simulink model "genericEE"  (R2021a)
settings: Solver=ode8  StartTime=0.0  StopTime=inf  FixedStep=0.001  RelTol=1e-3  EnableMultiTasking=on
StartFcn:
  | addpath('C:\Stud\Mgr_work\casadi-windows-matlabR2016a-v3.5.5')
  | import casadi.*
libraries: CarMaker4SL x35, simulink x1
(part 2 of 3)

== system genericEE/CarMaker/IPG Vehicle/CarAndTrailer/Forces/Tires ==
  note: The TireXX_Out signals will only be used if FileIdent is "CarMaker-Tire-CM4SL" in the tire parameter file!
      | An example parameter file can be found in Data/Tire/DT_CM4SL_UserTire.
  Sync_In : Inport
  TireFL_In : Inport  Port=2
  TireFR_In : Inport  Port=3
  TireRL_In : Inport  Port=4
  TireRR_In : Inport  Port=5
  Bus Creator{1..4} (4 alike) : BusCreator  Inputs=11
  Demux{1..3,8} (4 alike) : Demux  Outputs=7
      settings: DisplayOption=none
  TireFL : Subsystem
  TireFR : Subsystem
  TireRL : Subsystem
  TireRR : Subsystem
  TireFL_Out : Outport
  TireFR_Out : Outport  Port=2
  TireRL_Out : Outport  Port=3
  TireRR_Out : Outport  Port=4
  wires:
  Sync_In/1 -> TireRR/1(Sync_In), TireRL/1(Sync_In), TireFR/1(Sync_In), TireFL/1(Sync_In)
  Bus Creator4/1 -> TireRR_Out/1
  Bus Creator2/1 -> TireRL_Out/1
  Bus Creator1/1 -> TireFR_Out/1
  Demux3/5 -> TireRR/6(Rim_turnv)  "Tire_In Rim_turnv"
  Demux3/4 -> TireRR/5(Rim_rotv)  "Tire_In Rim_rotv"
  Demux3/1 -> TireRR/2(Load)  "Tire_In Load"
  Demux3/7 -> TireRR/8(muRoad)  "Tire_In mu"
  Demux3/6 -> TireRR/7(InclinAngle)  "Tire_In Camber"
  Demux3/2 -> TireRR/3(vxtrans)  "Tire_In vxtrans"
  Demux3/3 -> TireRR/4(vytrans)  "Tire_In vytrans"
  TireRR/11(AlignTrq) -> Bus Creator4/11  "Tire_Out AlignTrq"
  TireRR/10(RollResist) -> Bus Creator4/10  "Tire_Out RollResist"
  TireRR/9(OverturnTrq) -> Bus Creator4/9  "Tire_Out OverturnTrq"
  TireRR/8(LoadFrc) -> Bus Creator4/8  "Tire_Out LoadFrc"
  TireRR/7(SideFrc) -> Bus Creator4/7  "Tire_Out SideFrc"
  TireRR/6(LongFrc) -> Bus Creator4/6  "Tire_Out LongFrc"
  TireRR/5(vBelt) -> Bus Creator4/5  "Tire_Out vBelt"
  TireRR/4(rBelt_eff) -> Bus Creator4/4  "Tire_Out rBelt_eff"
  TireRR/3(TurnSlp) -> Bus Creator4/3  "Tire_Out TurnSlp"
  TireRR/1(Slp) -> Bus Creator4/1  "Tire_Out Slp"
  TireRR/2(Alpha) -> Bus Creator4/2  "Tire_Out Alpha"
  Demux2/5 -> TireRL/6(Rim_turnv)  "Tire_In Rim_turnv"
  Demux2/4 -> TireRL/5(Rim_rotv)  "Tire_In Rim_rotv"
  Demux2/1 -> TireRL/2(Load)  "Tire_In Load"
  Demux2/7 -> TireRL/8(muRoad)  "Tire_In mu"
  Demux2/6 -> TireRL/7(InclinAngle)  "Tire_In Camber"
  Demux2/2 -> TireRL/3(vxtrans)  "Tire_In vxtrans"
  Demux2/3 -> TireRL/4(vytrans)  "Tire_In vytrans"
  TireRL/11(AlignTrq) -> Bus Creator2/11  "Tire_Out AlignTrq"
  TireRL/10(RollResist) -> Bus Creator2/10  "Tire_Out RollResist"
  TireRL/9(OverturnTrq) -> Bus Creator2/9  "Tire_Out OverturnTrq"
  TireRL/8(LoadFrc) -> Bus Creator2/8  "Tire_Out LoadFrc"
  TireRL/7(SideFrc) -> Bus Creator2/7  "Tire_Out SideFrc"
  TireRL/6(LongFrc) -> Bus Creator2/6  "Tire_Out LongFrc"
  TireRL/5(vBelt) -> Bus Creator2/5  "Tire_Out vBelt"
  TireRL/4(rBelt_eff) -> Bus Creator2/4  "Tire_Out rBelt_eff"
  TireRL/3(TurnSlp) -> Bus Creator2/3  "Tire_Out TurnSlp"
  TireRL/1(Slp) -> Bus Creator2/1  "Tire_Out Slp"
  TireRL/2(Alpha) -> Bus Creator2/2  "Tire_Out Alpha"
  Demux1/5 -> TireFR/6(Rim_turnv)  "Tire_In Rim_turnv"
  Demux1/4 -> TireFR/5(Rim_rotv)  "Tire_In Rim_rotv"
  Demux1/1 -> TireFR/2(Load)  "Tire_In Load"
  Demux1/7 -> TireFR/8(muRoad)  "Tire_In mu"
  Demux1/6 -> TireFR/7(InclinAngle)  "Tire_In Camber"
  Demux1/2 -> TireFR/3(vxtrans)  "Tire_In vxtrans"
  Demux1/3 -> TireFR/4(vytrans)  "Tire_In vytrans"
  TireFR/11(AlignTrq) -> Bus Creator1/11  "Tire_Out AlignTrq"
  TireFR/10(RollResist) -> Bus Creator1/10  "Tire_Out RollResist"
  TireFR/9(OverturnTrq) -> Bus Creator1/9  "Tire_Out OverturnTrq"
  TireFR/8(LoadFrc) -> Bus Creator1/8  "Tire_Out LoadFrc"
  TireFR/7(SideFrc) -> Bus Creator1/7  "Tire_Out SideFrc"
  TireFR/6(LongFrc) -> Bus Creator1/6  "Tire_Out LongFrc"
  TireFR/5(vBelt) -> Bus Creator1/5  "Tire_Out vBelt"
  TireFR/4(rBelt_eff) -> Bus Creator1/4  "Tire_Out rBelt_eff"
  TireFR/3(TurnSlp) -> Bus Creator1/3  "Tire_Out TurnSlp"
  TireFR/1(Slp) -> Bus Creator1/1  "Tire_Out Slp"
  TireFR/2(Alpha) -> Bus Creator1/2  "Tire_Out Alpha"
  Demux8/5 -> TireFL/6(Rim_turnv)  "Tire_In Rim_turnv"
  Demux8/4 -> TireFL/5(Rim_rotv)  "Tire_In Rim_rotv"
  TireFL_In/1 -> Demux8/1
  Demux8/1 -> TireFL/2(Load)  "Tire_In Load"
  Demux8/7 -> TireFL/8(muRoad)  "Tire_In mu"
  Demux8/6 -> TireFL/7(InclinAngle)  "Tire_In Camber"
  Demux8/2 -> TireFL/3(vxtrans)  "Tire_In vxtrans"
  Demux8/3 -> TireFL/4(vytrans)  "Tire_In vytrans"
  TireFL/11(AlignTrq) -> Bus Creator3/11  "Tire_Out AlignTrq"
  TireFL/10(RollResist) -> Bus Creator3/10  "Tire_Out RollResist"
  TireFL/9(OverturnTrq) -> Bus Creator3/9  "Tire_Out OverturnTrq"
  TireFL/8(LoadFrc) -> Bus Creator3/8  "Tire_Out LoadFrc"
  TireFL/7(SideFrc) -> Bus Creator3/7  "Tire_Out SideFrc"
  TireFL/6(LongFrc) -> Bus Creator3/6  "Tire_Out LongFrc"
  TireFL/5(vBelt) -> Bus Creator3/5  "Tire_Out vBelt"
  TireFL/4(rBelt_eff) -> Bus Creator3/4  "Tire_Out rBelt_eff"
  TireFL/3(TurnSlp) -> Bus Creator3/3  "Tire_Out TurnSlp"
  TireFL/1(Slp) -> Bus Creator3/1  "Tire_Out Slp"
  TireFL/2(Alpha) -> Bus Creator3/2  "Tire_Out Alpha"
  Bus Creator3/1 -> TireFL_Out/1
  TireFR_In/1 -> Demux1/1
  TireRL_In/1 -> Demux2/1
  TireRR_In/1 -> Demux3/1

== system genericEE/CarMaker/IPG Vehicle/CarAndTrailer/Forces/Vehicle Forces ==
  Sync_In : Inport
  Bus Creator1 : BusCreator  Inputs=12
  Bus Creator8 : BusCreator  Inputs=16
  BusCreator1 : BusCreator  Inputs=4
  BusCreator2 : BusCreator  Inputs=9
  Demux : Demux  Outputs=16
      settings: DisplayOption=none
  Demux1 : Demux  Outputs=12
      settings: DisplayOption=none
  Demux2 : Demux  Outputs=13
      settings: DisplayOption=none
  Forces : S-Function  FunctionName=CM_Sfun  Parameters='Forces'  SFunctionDeploymentMode=off  EnableBusSupport=off
  Terminator : Terminator
  Sync_Out : Outport
  Car.Virtual : Outport  Port=2
  Car.Aero : Outport  Port=3
  Car.Load : Outport  Port=4
  wires:
  BusCreator1/1 -> Terminator/1  "Aero IF (in)"
  Demux2/13 -> BusCreator2/9  "car Aero Trq_1 z"
  Demux2/12 -> BusCreator2/8  "car Aero Trq_1 y"
  Demux2/11 -> BusCreator2/7  "car Aero Trq_1 x"
  Demux2/10 -> BusCreator2/6  "car Aero Frc_1 z"
  Demux2/9 -> BusCreator2/5  "car Aero Frc_1 y"
  Demux2/8 -> BusCreator2/4  "car Aero Frc_1 x"
  Demux2/7 -> BusCreator2/3  "car Aero PoA_1 z"
  Demux2/6 -> BusCreator2/2  "car Aero PoA_1 y"
  Demux2/5 -> BusCreator2/1  "car Aero PoA_1 x"
  Demux2/4 -> BusCreator1/4  "car Aero tau_1"
  Demux2/3 -> BusCreator1/3  "car Aero ApproachVel_1 z"
  Demux2/2 -> BusCreator1/2  "car Aero ApproachVel_1 y"
  Demux2/1 -> BusCreator1/1  "car Aero ApproachVel_1 x"
  Demux/16 -> Bus Creator8/16  "Car Load_3 tz"
  Demux/15 -> Bus Creator8/15  "Car Load_3 ty"
  Demux/14 -> Bus Creator8/14  "Car Load_3 tx"
  Demux/13 -> Bus Creator8/13  "Car Load_3 mass"
  Demux1/12 -> Bus Creator1/12  "Car Virtual Trq_0 z"
  Demux1/11 -> Bus Creator1/11  "Car Virtual Trq_0 y"
  Demux1/10 -> Bus Creator1/10  "Car Virtual Trq_0 x"
  Demux1/9 -> Bus Creator1/9  "Car Virtual Trq_1 z"
  Demux1/8 -> Bus Creator1/8  "Car Virtual Trq_1 y"
  Demux1/7 -> Bus Creator1/7  "Car Virtual Trq_1 x"
  Demux1/6 -> Bus Creator1/6  "Car Virtual Frc_0 z"
  Demux1/5 -> Bus Creator1/5  "Car Virtual Frc_0 y"
  Demux1/4 -> Bus Creator1/4  "Car Virtual Frc_0 x"
  Sync_In/1 -> Forces/1
  Forces/1 -> Sync_Out/1
  BusCreator2/1 -> Car.Aero/1
  Demux1/1 -> Bus Creator1/1  "Car Virtual Frc_1 x"
  Demux1/2 -> Bus Creator1/2  "Car Virtual Frc_1 y"
  Demux1/3 -> Bus Creator1/3  "Car Virtual Frc_1 z"
  Forces/3 -> Demux2/1
  Forces/2 -> Demux1/1
  Bus Creator1/1 -> Car.Virtual/1
  Bus Creator8/1 -> Car.Load/1
  Demux/1 -> Bus Creator8/1  "Car Load_0 mass"
  Demux/2 -> Bus Creator8/2  "Car Load_0 tx"
  Demux/3 -> Bus Creator8/3  "Car Load_0 ty"
  Demux/4 -> Bus Creator8/4  "Car Load_0 tz"
  Demux/5 -> Bus Creator8/5  "Car Load_1 mass"
  Demux/6 -> Bus Creator8/6  "Car Load_1 tx"
  Demux/7 -> Bus Creator8/7  "Car Load_1 ty"
  Demux/8 -> Bus Creator8/8  "Car Load_1 tz"
  Demux/9 -> Bus Creator8/9  "Car Load_2 mass"
  Demux/10 -> Bus Creator8/10  "Car Load_2 tx"
  Demux/11 -> Bus Creator8/11  "Car Load_2 ty"
  Demux/12 -> Bus Creator8/12  "Car Load_2 tz"
  Forces/4 -> Demux/1

== system genericEE/CarMaker/IPG Vehicle/CarAndTrailer/Trailer/CreateBus Car.Hitch.FrcTrq ==
  In1 : Inport
  Bus Creator7 : BusCreator  Inputs=6
  Demux7 : Demux  Outputs=6
      settings: DisplayOption=none
  Out1 : Outport
  wires:
  In1/1 -> Demux7/1
  Bus Creator7/1 -> Out1/1
  Demux7/6 -> Bus Creator7/6  "Car Hitch Trq2Car z"
  Demux7/5 -> Bus Creator7/5  "Car Hitch Trq2Car y"
  Demux7/4 -> Bus Creator7/4  "Car Hitch Trq2Car x"
  Demux7/3 -> Bus Creator7/3  "Car Hitch Frc2Car z"
  Demux7/2 -> Bus Creator7/2  "Car Hitch Frc2Car y"
  Demux7/1 -> Bus Creator7/1  "Car Hitch Frc2Car x"

== system genericEE/CarMaker/IPG Vehicle/CarAndTrailer/Trailer/CreateBus Vhcl.Motion ==
  In1 : Inport
  BusCreator : BusCreator  Inputs=15
  Demux : Demux  Outputs=15
      settings: DisplayOption=none
  Out1 : Outport
  wires:
  Demux/15 -> BusCreator/15  "Vhcl YawAcc"
  Demux/14 -> BusCreator/14  "Vhcl YawVel"
  Demux/13 -> BusCreator/13  "Vhcl Yaw"
  Demux/12 -> BusCreator/12  "Vhcl PitchAcc"
  Demux/11 -> BusCreator/11  "Vhcl PitchVel"
  Demux/10 -> BusCreator/10  "Vhcl Pitch"
  Demux/9 -> BusCreator/9  "Vhcl RollAcc"
  Demux/8 -> BusCreator/8  "Vhcl RollVel"
  Demux/7 -> BusCreator/7  "Vhcl Roll"
  Demux/6 -> BusCreator/6  "Vhcl Hitch_Pos z"
  Demux/5 -> BusCreator/5  "Vhcl Hitch_Pos y"
  Demux/4 -> BusCreator/4  "Vhcl Hitch_Pos x"
  Demux/3 -> BusCreator/3  "Vhcl sRoad"
  Demux/2 -> BusCreator/2  "Vhcl Distance"
  Demux/1 -> BusCreator/1  "Vhcl v"
  In1/1 -> Demux/1
  BusCreator/1 -> Out1/1

== system genericEE/CarMaker/IPG Vehicle/CarAndTrailer/Trailer/CreateBus Vhcl.PoI ==
  In1 : Inport
  Bus Creator3 : BusCreator  Inputs=18
  Demux3 : Demux  Outputs=18
      settings: DisplayOption=none
  Out1 : Outport
  wires:
  Demux3/18 -> Bus Creator3/18  "Vhcl PoI_GCS Elev"
  Demux3/17 -> Bus Creator3/17  "Vhcl PoI_GCS Lat"
  Demux3/16 -> Bus Creator3/16  "Vhcl PoI_GCS Long"
  Demux3/15 -> Bus Creator3/15  "Vhcl PoI_Acc_1 z"
  Demux3/14 -> Bus Creator3/14  "Vhcl PoI_Acc_1 y"
  Demux3/13 -> Bus Creator3/13  "Vhcl PoI_Acc_1 x"
  Demux3/12 -> Bus Creator3/12  "Vhcl PoI_Vel_1 z"
  Demux3/11 -> Bus Creator3/11  "Vhcl PoI_Vel_1 y"
  Demux3/10 -> Bus Creator3/10  "Vhcl PoI_Vel_1 x"
  Demux3/9 -> Bus Creator3/9  "Vhcl PoI_Acc z"
  Demux3/8 -> Bus Creator3/8  "Vhcl PoI_Acc y"
  Demux3/7 -> Bus Creator3/7  "Vhcl PoI_Acc x"
  Demux3/6 -> Bus Creator3/6  "Vhcl PoI_Vel z"
  Demux3/5 -> Bus Creator3/5  "Vhcl PoI_Vel y"
  Demux3/4 -> Bus Creator3/4  "Vhcl PoI_Vel x"
  Demux3/3 -> Bus Creator3/3  "Vhcl PoI_Pos z"
  Demux3/2 -> Bus Creator3/2  "Vhcl PoI_Pos y"
  In1/1 -> Demux3/1
  Bus Creator3/1 -> Out1/1
  Demux3/1 -> Bus Creator3/1  "Vhcl PoI_Pos x"

== system genericEE/CarMaker/IPG Vehicle/CarAndTrailer/Trailer/CreateBus Vhcl.Steering ==
  In1 : Inport
  Bus Creator3 : BusCreator  Inputs=4
  Demux : Demux
      settings: DisplayOption=none
  Out1 : Outport
  wires:
  Bus Creator3/1 -> Out1/1
  Demux/1 -> Bus Creator3/1  "Vhcl Steering Ang"
  Demux/3 -> Bus Creator3/3  "Vhcl Steering AngAcc"
  Demux/2 -> Bus Creator3/2  "Vhcl Steering AngVel"
  Demux/4 -> Bus Creator3/4  "Vhcl Steering Trq"
  In1/1 -> Demux/1

== system genericEE/CarMaker/IPG Vehicle/CarAndTrailer/Trailer/CreateBus Vhcl.Wheel.FL ==
  In1 : Inport
  Bus Creator3 : BusCreator  Inputs=14
  Demux3 : Demux  Outputs=14
      settings: DisplayOption=none
  Out1 : Outport
  wires:
  Demux3/14 -> Bus Creator3/14  "Vhcl Wheel FL Trq_WhlBearing"
  Demux3/13 -> Bus Creator3/13  "Vhcl Wheel FL Trq_T2W"
  Demux3/12 -> Bus Creator3/12  "Vhcl Wheel FL SideSlip"
  Demux3/11 -> Bus Creator3/11  "Vhcl Wheel FL LongSlip"
  Demux3/10 -> Bus Creator3/10  "Vhcl Wheel FL vBelt"
  Demux3/9 -> Bus Creator3/9  "Vhcl Wheel FL Fz"
  Demux3/8 -> Bus Creator3/8  "Vhcl Wheel FL Fy"
  Demux3/7 -> Bus Creator3/7  "Vhcl Wheel FL Fx"
  Demux3/6 -> Bus Creator3/6  "Vhcl Wheel FL r_zxy z"
  Demux3/5 -> Bus Creator3/5  "Vhcl Wheel FL r_zxy y"
  Demux3/4 -> Bus Creator3/4  "Vhcl Wheel FL r_zxy x"
  Demux3/3 -> Bus Creator3/3  "Vhcl Wheel FL t z"
  Demux3/2 -> Bus Creator3/2  "Vhcl Wheel FL t y"
  In1/1 -> Demux3/1
  Bus Creator3/1 -> Out1/1
  Demux3/1 -> Bus Creator3/1  "Vhcl Wheel FL t x"

== system genericEE/CarMaker/IPG Vehicle/CarAndTrailer/Trailer/CreateBus Vhcl.Wheel.FR ==
  In1 : Inport
  Bus Creator3 : BusCreator  Inputs=14
  Demux3 : Demux  Outputs=14
      settings: DisplayOption=none
  Out1 : Outport
  wires:
  Demux3/14 -> Bus Creator3/14  "Vhcl Wheel FR Trq_WhlBearing"
  Demux3/13 -> Bus Creator3/13  "Vhcl Wheel FR Trq_T2W"
  Demux3/12 -> Bus Creator3/12  "Vhcl Wheel FR SideSlip"
  Demux3/11 -> Bus Creator3/11  "Vhcl Wheel FR LongSlip"
  Demux3/10 -> Bus Creator3/10  "Vhcl Wheel FR vBelt"
  Demux3/9 -> Bus Creator3/9  "Vhcl Wheel FR Fz"
  Demux3/8 -> Bus Creator3/8  "Vhcl Wheel FR Fy"
  Demux3/7 -> Bus Creator3/7  "Vhcl Wheel FR Fx"
  Demux3/6 -> Bus Creator3/6  "Vhcl Wheel FR r_zxy z"
  Demux3/5 -> Bus Creator3/5  "Vhcl Wheel FR r_zxy y"
  Demux3/4 -> Bus Creator3/4  "Vhcl Wheel FR r_zxy x"
  Demux3/3 -> Bus Creator3/3  "Vhcl Wheel FR t z"
  Demux3/2 -> Bus Creator3/2  "Vhcl Wheel FR t y"
  In1/1 -> Demux3/1
  Bus Creator3/1 -> Out1/1
  Demux3/1 -> Bus Creator3/1  "Vhcl Wheel FR t x"

== system genericEE/CarMaker/IPG Vehicle/CarAndTrailer/Trailer/CreateBus Vhcl.Wheel.RL ==
  In1 : Inport
  Bus Creator3 : BusCreator  Inputs=14
  Demux3 : Demux  Outputs=14
      settings: DisplayOption=none
  Out1 : Outport
  wires:
  Demux3/14 -> Bus Creator3/14  "Vhcl Wheel RL Trq_WhlBearing"
  Demux3/13 -> Bus Creator3/13  "Vhcl Wheel RL Trq_T2W"
  Demux3/12 -> Bus Creator3/12  "Vhcl Wheel RL SideSlip"
  Demux3/11 -> Bus Creator3/11  "Vhcl Wheel RL LongSlip"
  Demux3/10 -> Bus Creator3/10  "Vhcl Wheel RL vBelt"
  Demux3/9 -> Bus Creator3/9  "Vhcl Wheel RL Fz"
  Demux3/8 -> Bus Creator3/8  "Vhcl Wheel RL Fy"
  Demux3/7 -> Bus Creator3/7  "Vhcl Wheel RL Fx"
  Demux3/6 -> Bus Creator3/6  "Vhcl Wheel RL r_zxy z"
  Demux3/5 -> Bus Creator3/5  "Vhcl Wheel RL r_zxy y"
  Demux3/4 -> Bus Creator3/4  "Vhcl Wheel RL r_zxy x"
  Demux3/3 -> Bus Creator3/3  "Vhcl Wheel RL t z"
  Demux3/2 -> Bus Creator3/2  "Vhcl Wheel RL t y"
  In1/1 -> Demux3/1
  Bus Creator3/1 -> Out1/1
  Demux3/1 -> Bus Creator3/1  "Vhcl Wheel RL t x"

== system genericEE/CarMaker/IPG Vehicle/CarAndTrailer/Trailer/CreateBus Vhcl.Wheel.RR ==
  In1 : Inport
  Bus Creator3 : BusCreator  Inputs=14
  Demux3 : Demux  Outputs=14
      settings: DisplayOption=none
  Out1 : Outport
  wires:
  Demux3/14 -> Bus Creator3/14  "Vhcl Wheel RR Trq_WhlBearing"
  Demux3/13 -> Bus Creator3/13  "Vhcl Wheel RR Trq_T2W"
  Demux3/12 -> Bus Creator3/12  "Vhcl Wheel RR SideSlip"
  Demux3/11 -> Bus Creator3/11  "Vhcl Wheel RR LongSlip"
  Demux3/10 -> Bus Creator3/10  "Vhcl Wheel RR vBelt"
  Demux3/9 -> Bus Creator3/9  "Vhcl Wheel RR Fz"
  Demux3/8 -> Bus Creator3/8  "Vhcl Wheel RR Fy"
  Demux3/7 -> Bus Creator3/7  "Vhcl Wheel RR Fx"
  Demux3/6 -> Bus Creator3/6  "Vhcl Wheel RR r_zxy z"
  Demux3/5 -> Bus Creator3/5  "Vhcl Wheel RR r_zxy y"
  Demux3/4 -> Bus Creator3/4  "Vhcl Wheel RR r_zxy x"
  Demux3/3 -> Bus Creator3/3  "Vhcl Wheel RR t z"
  Demux3/2 -> Bus Creator3/2  "Vhcl Wheel RR t y"
  In1/1 -> Demux3/1
  Bus Creator3/1 -> Out1/1
  Demux3/1 -> Bus Creator3/1  "Vhcl Wheel RR t x"

== system genericEE/CarMaker/VehicleControl/CreateBus VhclCtrl/Environmental Envelope Protection/Control switcher with memory ==
  v : Inport
  thr : Inport  Port=2
  Integrator : Integrator  LimitOutput=on  UpperSaturationLimit=0.2  LowerSaturationLimit=-0.2
  MATLAB Function : MATLAB Function  TreatAsAtomicUnit=on
  Scope : Scope  NumInputPorts=2
  Sign : Signum
  control_flag : Outport
  wires:
  Sign/1 -> control_flag/1
  MATLAB Function/1(control_on) -> Scope/1, Integrator/1
  thr/1 -> MATLAB Function/2(thr)
  Integrator/1 -> Scope/2, Sign/1
  v/1 -> MATLAB Function/1(v)

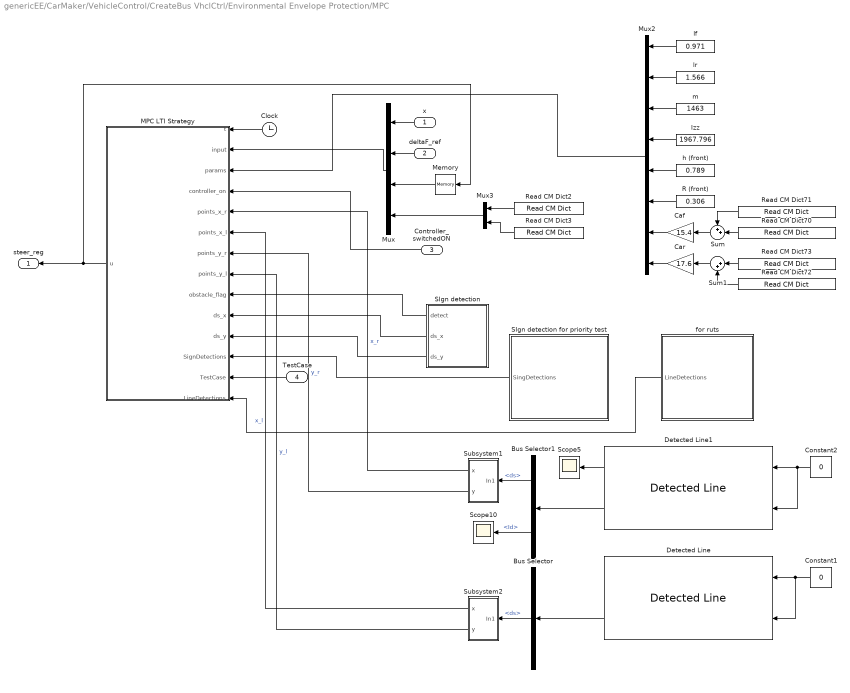
== system genericEE/CarMaker/VehicleControl/CreateBus VhclCtrl/Environmental Envelope Protection/MPC ==
  x : Inport
  deltaF_ref : Inport  Port=2
  Controller_switchedON : Inport  Port=3
  TestCase : Inport  Port=4
  Bus Selector : BusSelector  OutputSignals=ds
  Bus Selector1 : BusSelector  OutputSignals=ds,Id
  Caf : Gain  Gain=15.4
  Car : Gain  Gain=17.6
  Clock : Clock
  Constant1 : Constant  Value=0
  Constant2 : Constant  Value=0
  Detected Line : CarMaker4SL/Sensors/Detected Line  xname=INPORT  xstime=Continuous  xside=left
      settings: SourceProductName=CarMaker4SL
  Detected Line1 : CarMaker4SL/Sensors/Detected Line  xname=INPORT  xstime=Continuous  xside=right
      settings: SourceProductName=CarMaker4SL
  Izz : Constant  Value=1967.796
  MPC LTI Strategy : MATLAB Function  TreatAsAtomicUnit=on  SystemSampleTime=0.05
  Memory : Memory
  Mux : Mux
  Mux2 : Mux  Inputs=8
  Mux3 : Mux  Inputs=2
  R (front) : Constant  Value=0.306
  Read CM Dict2 : CarMaker4SL/Read CM Dict  xname=Car.tx  xsync=off  xstime=Continuous
  Read CM Dict3 : CarMaker4SL/Read CM Dict  xname=Car.ty  xsync=off  xstime=Continuous
  Read CM Dict70 : CarMaker4SL/Read CM Dict  xname=Vhcl.FL.Fz  xsync=off  xstime=Continuous
  Read CM Dict71 : CarMaker4SL/Read CM Dict  xname=Vhcl.FR.Fz  xsync=off  xstime=Continuous
  Read CM Dict72 : CarMaker4SL/Read CM Dict  xname=Vhcl.RL.Fz  xsync=off  xstime=Continuous
  Read CM Dict73 : CarMaker4SL/Read CM Dict  xname=Vhcl.RR.Fz  xsync=off  xstime=Continuous
  SIgn detection : Subsystem
  SIgn detection for priority test : Subsystem
  Scope10 : Scope
  Scope5 : Scope
  Subsystem1 : Subsystem
  Subsystem2 : Subsystem
  Sum : Sum  Inputs=++|
  Sum1 : Sum  Inputs=|++
  for ruts : Subsystem
  h (front) : Constant  Value=0.789
  lf : Constant  Value=0.971
  lr : Constant  Value=1.566
  m : Constant  Value=1463
  steer_reg : Outport  VectorParamsAs1DForOutWhenUnconnected=off
  wires:
  Mux/1 -> MPC LTI Strategy/2(input)
  deltaF_ref/1 -> Mux/2
  x/1 -> Mux/1
  Clock/1 -> MPC LTI Strategy/1(t)
  h (front)/1 -> Mux2/5
  R (front)/1 -> Mux2/6
  Mux2/1 -> MPC LTI Strategy/3(params)
  Izz/1 -> Mux2/4
  m/1 -> Mux2/3
  lr/1 -> Mux2/2
  lf/1 -> Mux2/1
  Read CM Dict71/1 -> Sum/1
  Read CM Dict70/1 -> Sum/2
  Sum/1 -> Caf/1
  Caf/1 -> Mux2/7
  Read CM Dict73/1 -> Sum1/1
  Sum1/1 -> Car/1
  Read CM Dict72/1 -> Sum1/2
  Car/1 -> Mux2/8
  Controller_switchedON/1 -> MPC LTI Strategy/4(controller_on)
  Memory/1 -> Mux/3
  Subsystem1/1(x) -> MPC LTI Strategy/5(points_x_r)  "x_r"
  Subsystem1/2(y) -> MPC LTI Strategy/7(points_y_r)  "y_r"
  Subsystem2/2(y) -> MPC LTI Strategy/8(points_y_l)  "y_l"
  Detected Line/2 -> Bus Selector/1
  Constant2/1 -> Detected Line1/2, Detected Line1/1
  Bus Selector1/1 -> Subsystem1/1(In1)  "<ds>"
  Subsystem2/1(x) -> MPC LTI Strategy/6(points_x_l)  "x_l"
  Constant1/1 -> Detected Line/2, Detected Line/1
  Bus Selector/1 -> Subsystem2/1(In1)  "<ds>"
  Detected Line1/2 -> Bus Selector1/1
  Read CM Dict2/1 -> Mux3/1
  Read CM Dict3/1 -> Mux3/2
  Mux3/1 -> Mux/4
  SIgn detection/1(detect) -> MPC LTI Strategy/9(obstacle_flag)
  SIgn detection/3(ds_y) -> MPC LTI Strategy/11(ds_y)
  SIgn detection/2(ds_x) -> MPC LTI Strategy/10(ds_x)
  Detected Line1/1 -> Scope5/1
  Bus Selector1/2 -> Scope10/1  "<Id>"
  SIgn detection for priority test/1(SingDetections) -> MPC LTI Strategy/12(SignDetections)
  TestCase/1 -> MPC LTI Strategy/13(TestCase)
  for ruts/1(LineDetections) -> MPC LTI Strategy/14(LineDetections)
  MPC LTI Strategy/1(u) -> steer_reg/1, Memory/1

== system genericEE/CarMaker/VehicleControl/CreateBus VhclCtrl/Environmental Envelope Protection/Reference Generator ==
  Clock : Clock
  Clock2 : Clock
  Constant1 : Constant  Value=0
  Gain3 : Gain  Gain=0.1
  Gain4 : Gain  Gain=0.3
  Rate Limiter : RateLimiter  RisingSlewLimit=0.3  FallingSlewLimit=-0.3  SampleTimeMode=inherited
  Sin : Trigonometry
  Switch : Switch  Criteria=u2 > Threshold  Threshold=30
  Out1 : Outport
  wires:
  Clock2/1 -> Gain4/1
  Gain4/1 -> Sin/1
  Rate Limiter/1 -> Out1/1
  Switch/1 -> Rate Limiter/1
  Clock/1 -> Switch/2
  Sin/1 -> Gain3/1
  Gain3/1 -> Switch/3
  Constant1/1 -> Switch/1

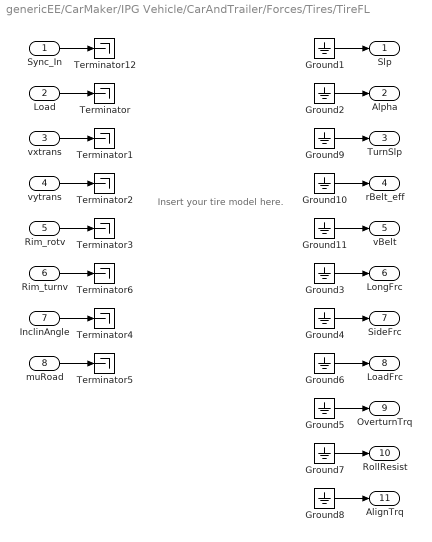
== system genericEE/CarMaker/IPG Vehicle/CarAndTrailer/Forces/Tires/TireFL ==
  note: Insert your tire model here.
  Sync_In : Inport
  Load : Inport  Port=2
  vxtrans : Inport  Port=3
  vytrans : Inport  Port=4
  Rim_rotv : Inport  Port=5
  Rim_turnv : Inport  Port=6
  InclinAngle : Inport  Port=7
  muRoad : Inport  Port=8
  Ground{1..11} (11 alike) : Ground
  Terminator{,1..6,12} (8 alike) : Terminator
  Slp : Outport
  Alpha : Outport  Port=2
  TurnSlp : Outport  Port=3
  rBelt_eff : Outport  Port=4
  vBelt : Outport  Port=5
  LongFrc : Outport  Port=6
  SideFrc : Outport  Port=7
  LoadFrc : Outport  Port=8
  OverturnTrq : Outport  Port=9
  RollResist : Outport  Port=10
  AlignTrq : Outport  Port=11
  wires:
  Ground11/1 -> vBelt/1
  Ground10/1 -> rBelt_eff/1
  Ground9/1 -> TurnSlp/1
  Rim_turnv/1 -> Terminator6/1
  Sync_In/1 -> Terminator12/1
  Ground2/1 -> Alpha/1
  Ground3/1 -> LongFrc/1
  Ground4/1 -> SideFrc/1
  Ground5/1 -> OverturnTrq/1
  vxtrans/1 -> Terminator1/1
  vytrans/1 -> Terminator2/1
  Rim_rotv/1 -> Terminator3/1
  InclinAngle/1 -> Terminator4/1
  muRoad/1 -> Terminator5/1
  Load/1 -> Terminator/1
  Ground1/1 -> Slp/1
  Ground6/1 -> LoadFrc/1
  Ground7/1 -> RollResist/1
  Ground8/1 -> AlignTrq/1

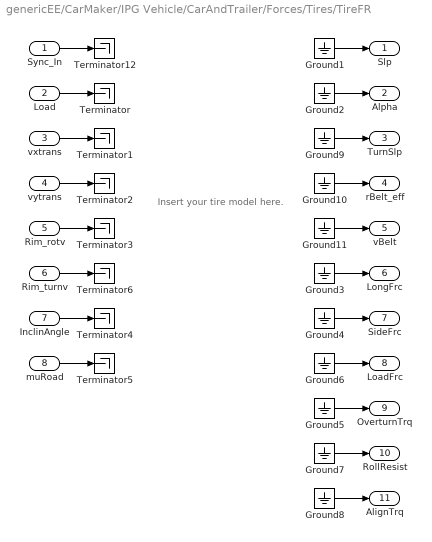
== system genericEE/CarMaker/IPG Vehicle/CarAndTrailer/Forces/Tires/TireFR ==
  note: Insert your tire model here.
  Sync_In : Inport
  Load : Inport  Port=2
  vxtrans : Inport  Port=3
  vytrans : Inport  Port=4
  Rim_rotv : Inport  Port=5
  Rim_turnv : Inport  Port=6
  InclinAngle : Inport  Port=7
  muRoad : Inport  Port=8
  Ground{1..11} (11 alike) : Ground
  Terminator{,1..6,12} (8 alike) : Terminator
  Slp : Outport
  Alpha : Outport  Port=2
  TurnSlp : Outport  Port=3
  rBelt_eff : Outport  Port=4
  vBelt : Outport  Port=5
  LongFrc : Outport  Port=6
  SideFrc : Outport  Port=7
  LoadFrc : Outport  Port=8
  OverturnTrq : Outport  Port=9
  RollResist : Outport  Port=10
  AlignTrq : Outport  Port=11
  wires:
  Ground11/1 -> vBelt/1
  Ground10/1 -> rBelt_eff/1
  Ground9/1 -> TurnSlp/1
  Rim_turnv/1 -> Terminator6/1
  Sync_In/1 -> Terminator12/1
  Ground2/1 -> Alpha/1
  Ground3/1 -> LongFrc/1
  Ground4/1 -> SideFrc/1
  Ground5/1 -> OverturnTrq/1
  vxtrans/1 -> Terminator1/1
  vytrans/1 -> Terminator2/1
  Rim_rotv/1 -> Terminator3/1
  InclinAngle/1 -> Terminator4/1
  muRoad/1 -> Terminator5/1
  Load/1 -> Terminator/1
  Ground1/1 -> Slp/1
  Ground6/1 -> LoadFrc/1
  Ground7/1 -> RollResist/1
  Ground8/1 -> AlignTrq/1

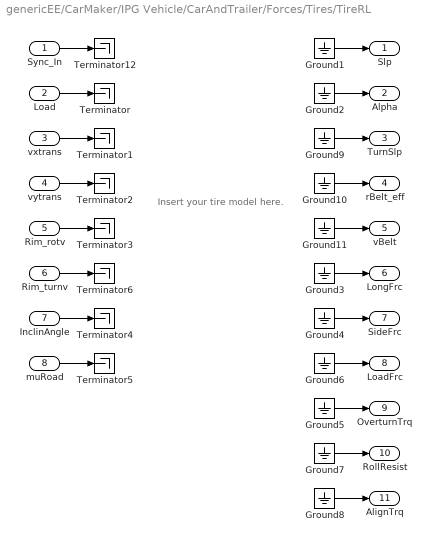
== system genericEE/CarMaker/IPG Vehicle/CarAndTrailer/Forces/Tires/TireRL ==
  note: Insert your tire model here.
  Sync_In : Inport
  Load : Inport  Port=2
  vxtrans : Inport  Port=3
  vytrans : Inport  Port=4
  Rim_rotv : Inport  Port=5
  Rim_turnv : Inport  Port=6
  InclinAngle : Inport  Port=7
  muRoad : Inport  Port=8
  Ground{1..11} (11 alike) : Ground
  Terminator{,1..6,12} (8 alike) : Terminator
  Slp : Outport
  Alpha : Outport  Port=2
  TurnSlp : Outport  Port=3
  rBelt_eff : Outport  Port=4
  vBelt : Outport  Port=5
  LongFrc : Outport  Port=6
  SideFrc : Outport  Port=7
  LoadFrc : Outport  Port=8
  OverturnTrq : Outport  Port=9
  RollResist : Outport  Port=10
  AlignTrq : Outport  Port=11
  wires:
  Ground11/1 -> vBelt/1
  Ground10/1 -> rBelt_eff/1
  Ground9/1 -> TurnSlp/1
  Rim_turnv/1 -> Terminator6/1
  Sync_In/1 -> Terminator12/1
  Ground2/1 -> Alpha/1
  Ground3/1 -> LongFrc/1
  Ground4/1 -> SideFrc/1
  Ground5/1 -> OverturnTrq/1
  vxtrans/1 -> Terminator1/1
  vytrans/1 -> Terminator2/1
  Rim_rotv/1 -> Terminator3/1
  InclinAngle/1 -> Terminator4/1
  muRoad/1 -> Terminator5/1
  Load/1 -> Terminator/1
  Ground1/1 -> Slp/1
  Ground6/1 -> LoadFrc/1
  Ground7/1 -> RollResist/1
  Ground8/1 -> AlignTrq/1

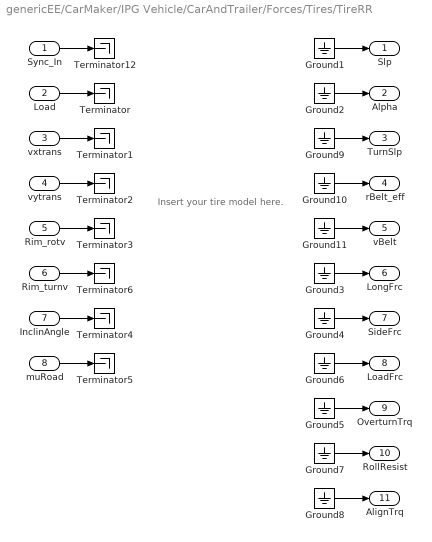
== system genericEE/CarMaker/IPG Vehicle/CarAndTrailer/Forces/Tires/TireRR ==
  note: Insert your tire model here.
  Sync_In : Inport
  Load : Inport  Port=2
  vxtrans : Inport  Port=3
  vytrans : Inport  Port=4
  Rim_rotv : Inport  Port=5
  Rim_turnv : Inport  Port=6
  InclinAngle : Inport  Port=7
  muRoad : Inport  Port=8
  Ground{1..11} (11 alike) : Ground
  Terminator{,1..6,12} (8 alike) : Terminator
  Slp : Outport
  Alpha : Outport  Port=2
  TurnSlp : Outport  Port=3
  rBelt_eff : Outport  Port=4
  vBelt : Outport  Port=5
  LongFrc : Outport  Port=6
  SideFrc : Outport  Port=7
  LoadFrc : Outport  Port=8
  OverturnTrq : Outport  Port=9
  RollResist : Outport  Port=10
  AlignTrq : Outport  Port=11
  wires:
  Ground11/1 -> vBelt/1
  Ground10/1 -> rBelt_eff/1
  Ground9/1 -> TurnSlp/1
  Rim_turnv/1 -> Terminator6/1
  Sync_In/1 -> Terminator12/1
  Ground2/1 -> Alpha/1
  Ground3/1 -> LongFrc/1
  Ground4/1 -> SideFrc/1
  Ground5/1 -> OverturnTrq/1
  vxtrans/1 -> Terminator1/1
  vytrans/1 -> Terminator2/1
  Rim_rotv/1 -> Terminator3/1
  InclinAngle/1 -> Terminator4/1
  muRoad/1 -> Terminator5/1
  Load/1 -> Terminator/1
  Ground1/1 -> Slp/1
  Ground6/1 -> LoadFrc/1
  Ground7/1 -> RollResist/1
  Ground8/1 -> AlignTrq/1

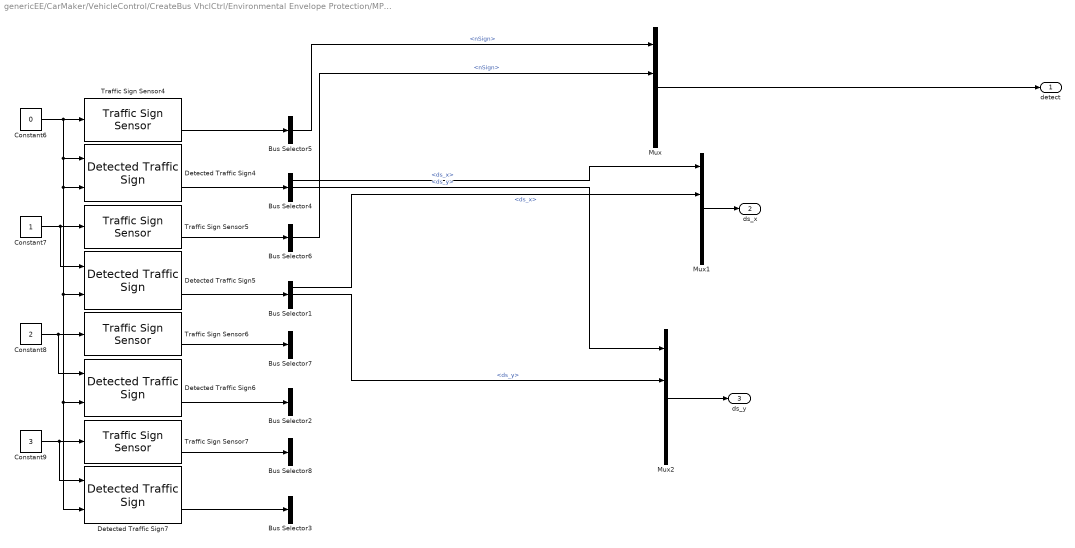
== system genericEE/CarMaker/VehicleControl/CreateBus VhclCtrl/Environmental Envelope Protection/MPC/SIgn detection ==
  Bus Selector1 : BusSelector  OutputSignals=ds_x,ds_y,ObjId
  Bus Selector2 : BusSelector  OutputSignals=ds_x,ds_y
  Bus Selector3 : BusSelector  OutputSignals=ds_x,ds_y
  Bus Selector4 : BusSelector  OutputSignals=ds_x,ds_y,ObjId
  Bus Selector{5..8} (4 alike) : BusSelector  OutputSignals=nSign
  Constant6 : Constant  Value=0
  Constant7 : Constant
  Constant8 : Constant  Value=2
  Constant9 : Constant  Value=3
  Detected Traffic Sign{4..7} (4 alike) : CarMaker4SL/Sensors/Detected Traffic Sign  xname=INPORT  xstime=Continuous
      settings: SourceProductName=CarMaker4SL
  Mux : Mux
  Mux1 : Mux
  Mux2 : Mux
  Traffic Sign Sensor{4..7} (4 alike) : CarMaker4SL/Sensors/Traffic Sign Sensor  xname=INPORT  xstime=Continuous
      settings: SourceProductName=CarMaker4SL
  detect : Outport
  ds_x : Outport  Port=2
  ds_y : Outport  Port=3
  wires:
  Traffic Sign Sensor4/2 -> Bus Selector5/1
  Constant7/1 -> Detected Traffic Sign5/1, Traffic Sign Sensor5/1
  Detected Traffic Sign4/2 -> Bus Selector4/1
  Detected Traffic Sign5/2 -> Bus Selector1/1
  Constant6/1 -> Detected Traffic Sign7/2, Detected Traffic Sign6/2, Detected Traffic Sign5/2, Detected Traffic Sign4/2, Detected Traffic Sign4/1, Traffic Sign Sensor4/1
  Constant8/1 -> Traffic Sign Sensor6/1, Detected Traffic Sign6/1
  Constant9/1 -> Traffic Sign Sensor7/1, Detected Traffic Sign7/1
  Traffic Sign Sensor5/2 -> Bus Selector6/1
  Detected Traffic Sign6/2 -> Bus Selector2/1
  Traffic Sign Sensor6/2 -> Bus Selector7/1
  Traffic Sign Sensor7/2 -> Bus Selector8/1
  Detected Traffic Sign7/2 -> Bus Selector3/1
  Mux1/1 -> ds_x/1
  Mux2/1 -> ds_y/1
  Mux/1 -> detect/1
  Bus Selector5/1 -> Mux/1  "<nSign>"
  Bus Selector6/1 -> Mux/2  "<nSign>"
  Bus Selector4/1 -> Mux1/1  "<ds_x>"
  Bus Selector1/1 -> Mux1/2  "<ds_x>"
  Bus Selector4/2 -> Mux2/1  "<ds_y>"
  Bus Selector1/2 -> Mux2/2  "<ds_y>"

== system genericEE/CarMaker/VehicleControl/CreateBus VhclCtrl/Environmental Envelope Protection/MPC/SIgn detection for priority test ==
  Bus Selector1 : BusSelector  OutputSignals=ds_x,ds_y,ObjId
  Bus Selector2 : BusSelector  OutputSignals=ds_x,ds_y,ObjId
  Bus Selector4 : BusSelector  OutputSignals=ds_x,ds_y,ObjId
  Constant : Constant  Value=11
  Constant1 : Constant  Value=13
  Constant6 : Constant  Value=0
  Constant7 : Constant
  Constant8 : Constant  Value=2
  Detected Traffic Sign4 : CarMaker4SL/Sensors/Detected Traffic Sign  xname=INPORT  xstime=Continuous
      settings: SourceProductName=CarMaker4SL
  Detected Traffic Sign5 : CarMaker4SL/Sensors/Detected Traffic Sign  xname=INPORT  xstime=Continuous
      settings: SourceProductName=CarMaker4SL
  Detected Traffic Sign6 : CarMaker4SL/Sensors/Detected Traffic Sign  xname=INPORT  xstime=Continuous
      settings: SourceProductName=CarMaker4SL
  MATLAB Function : MATLAB Function  TreatAsAtomicUnit=on
  MATLAB Function1 : MATLAB Function  TreatAsAtomicUnit=on
  Mux : Mux  Inputs=3
  Mux1 : Mux  Inputs=3
  Mux2 : Mux  Inputs=3
  Mux3 : Mux
  Scope4 : Scope
  SingDetections : Outport
  wires:
  Constant7/1 -> Detected Traffic Sign5/1
  Detected Traffic Sign4/2 -> Bus Selector4/1
  Detected Traffic Sign5/2 -> Bus Selector1/1
  Constant6/1 -> Detected Traffic Sign4/1, Detected Traffic Sign6/2, Detected Traffic Sign5/2, Detected Traffic Sign4/2
  Constant8/1 -> Detected Traffic Sign6/1
  Detected Traffic Sign6/2 -> Bus Selector2/1
  Bus Selector4/1 -> Mux1/1  "<ds_x>"
  Bus Selector1/1 -> Mux1/2  "<ds_x>"
  Bus Selector2/1 -> Mux1/3  "<ds_x>"
  Bus Selector4/3 -> Mux/1  "<ObjId>"
  Bus Selector1/3 -> Mux/2  "<ObjId>"
  Bus Selector2/3 -> Mux/3  "<ObjId>"
  Bus Selector4/2 -> Mux2/1  "<ds_y>"
  Bus Selector1/2 -> Mux2/2  "<ds_y>"
  Bus Selector2/2 -> Mux2/3  "<ds_y>"
  Mux/1 -> Scope4/1, MATLAB Function1/2(ids), MATLAB Function/2(ids)
  Mux1/1 -> MATLAB Function1/3(X), MATLAB Function/3(X)
  Mux2/1 -> MATLAB Function1/4(Y), MATLAB Function/4(Y)
  Constant/1 -> MATLAB Function/1(sing_id)
  MATLAB Function/1(point_x) -> Mux3/1
  MATLAB Function/2(point_y) -> Mux3/2
  Constant1/1 -> MATLAB Function1/1(sing_id)
  MATLAB Function1/1(point_x) -> Mux3/3
  MATLAB Function1/2(point_y) -> Mux3/4
  Mux3/1 -> SingDetections/1

== system genericEE/CarMaker/VehicleControl/CreateBus VhclCtrl/Environmental Envelope Protection/MPC/Subsystem1 ==
  In1 : Inport
  Bus Selector{1..10} (10 alike) : BusSelector  OutputSignals=x,y,z
  Mux : Mux  Inputs=10
  Mux1 : Mux  Inputs=10
  Selector1 : Selector  InputPortWidth=200  IndexOptions=Index vector (dialog)  Indices=1  OutputSizes=1
  Selector10 : Selector  InputPortWidth=200  IndexOptions=Index vector (dialog)  Indices=10  OutputSizes=1
  Selector2 : Selector  InputPortWidth=200  IndexOptions=Index vector (dialog)  Indices=2  OutputSizes=1
  Selector3 : Selector  InputPortWidth=200  IndexOptions=Index vector (dialog)  Indices=3  OutputSizes=1
  Selector4 : Selector  InputPortWidth=200  IndexOptions=Index vector (dialog)  Indices=4  OutputSizes=1
  Selector5 : Selector  InputPortWidth=200  IndexOptions=Index vector (dialog)  Indices=5  OutputSizes=1
  Selector6 : Selector  InputPortWidth=200  IndexOptions=Index vector (dialog)  Indices=6  OutputSizes=1
  Selector7 : Selector  InputPortWidth=200  IndexOptions=Index vector (dialog)  Indices=7  OutputSizes=1
  Selector8 : Selector  InputPortWidth=200  IndexOptions=Index vector (dialog)  Indices=8  OutputSizes=1
  Selector9 : Selector  InputPortWidth=200  IndexOptions=Index vector (dialog)  Indices=9  OutputSizes=1
  x : Outport
  y : Outport  Port=2
  wires:
  Bus Selector1/1 -> Mux/1  "<x>"
  Bus Selector2/2 -> Mux1/2  "<y>"
  In1/1 -> Selector2/1, Selector3/1, Selector4/1, Selector5/1, Selector6/1, Selector7/1, Selector8/1, Selector9/1, Selector10/1, Selector1/1
  Bus Selector2/1 -> Mux/2  "<x>"
  Selector2/1 -> Bus Selector2/1
  Selector1/1 -> Bus Selector1/1
  Bus Selector1/2 -> Mux1/1  "<y>"
  Bus Selector3/1 -> Mux/3  "<x>"
  Bus Selector3/2 -> Mux1/3  "<y>"
  Selector3/1 -> Bus Selector3/1
  Bus Selector4/1 -> Mux/4  "<x>"
  Bus Selector4/2 -> Mux1/4  "<y>"
  Selector4/1 -> Bus Selector4/1
  Bus Selector5/1 -> Mux/5  "<x>"
  Bus Selector5/2 -> Mux1/5  "<y>"
  Selector5/1 -> Bus Selector5/1
  Bus Selector6/1 -> Mux/6  "<x>"
  Bus Selector6/2 -> Mux1/6  "<y>"
  Selector6/1 -> Bus Selector6/1
  Bus Selector7/1 -> Mux/7  "<x>"
  Bus Selector7/2 -> Mux1/7  "<y>"
  Selector7/1 -> Bus Selector7/1
  Bus Selector8/1 -> Mux/8  "<x>"
  Bus Selector8/2 -> Mux1/8  "<y>"
  Selector8/1 -> Bus Selector8/1
  Bus Selector9/1 -> Mux/9  "<x>"
  Bus Selector9/2 -> Mux1/9  "<y>"
  Selector9/1 -> Bus Selector9/1
  Bus Selector10/1 -> Mux/10  "<x>"
  Bus Selector10/2 -> Mux1/10  "<y>"
  Selector10/1 -> Bus Selector10/1
  Mux/1 -> x/1
  Mux1/1 -> y/1

== system genericEE/CarMaker/VehicleControl/CreateBus VhclCtrl/Environmental Envelope Protection/MPC/Subsystem2 ==
  In1 : Inport
  Bus Selector{1..10} (10 alike) : BusSelector  OutputSignals=x,y,z
  Mux : Mux  Inputs=10
  Mux1 : Mux  Inputs=10
  Selector1 : Selector  InputPortWidth=200  IndexOptions=Index vector (dialog)  Indices=1  OutputSizes=1
  Selector10 : Selector  InputPortWidth=200  IndexOptions=Index vector (dialog)  Indices=10  OutputSizes=1
  Selector2 : Selector  InputPortWidth=200  IndexOptions=Index vector (dialog)  Indices=2  OutputSizes=1
  Selector3 : Selector  InputPortWidth=200  IndexOptions=Index vector (dialog)  Indices=3  OutputSizes=1
  Selector4 : Selector  InputPortWidth=200  IndexOptions=Index vector (dialog)  Indices=4  OutputSizes=1
  Selector5 : Selector  InputPortWidth=200  IndexOptions=Index vector (dialog)  Indices=5  OutputSizes=1
  Selector6 : Selector  InputPortWidth=200  IndexOptions=Index vector (dialog)  Indices=6  OutputSizes=1
  Selector7 : Selector  InputPortWidth=200  IndexOptions=Index vector (dialog)  Indices=7  OutputSizes=1
  Selector8 : Selector  InputPortWidth=200  IndexOptions=Index vector (dialog)  Indices=8  OutputSizes=1
  Selector9 : Selector  InputPortWidth=200  IndexOptions=Index vector (dialog)  Indices=9  OutputSizes=1
  x : Outport
  y : Outport  Port=2
  wires:
  Bus Selector1/1 -> Mux/1  "<x>"
  Bus Selector2/2 -> Mux1/2  "<y>"
  In1/1 -> Selector2/1, Selector3/1, Selector4/1, Selector5/1, Selector6/1, Selector7/1, Selector8/1, Selector9/1, Selector10/1, Selector1/1
  Bus Selector2/1 -> Mux/2  "<x>"
  Selector2/1 -> Bus Selector2/1
  Selector1/1 -> Bus Selector1/1
  Bus Selector1/2 -> Mux1/1  "<y>"
  Bus Selector3/1 -> Mux/3  "<x>"
  Bus Selector3/2 -> Mux1/3  "<y>"
  Selector3/1 -> Bus Selector3/1
  Bus Selector4/1 -> Mux/4  "<x>"
  Bus Selector4/2 -> Mux1/4  "<y>"
  Selector4/1 -> Bus Selector4/1
  Bus Selector5/1 -> Mux/5  "<x>"
  Bus Selector5/2 -> Mux1/5  "<y>"
  Selector5/1 -> Bus Selector5/1
  Bus Selector6/1 -> Mux/6  "<x>"
  Bus Selector6/2 -> Mux1/6  "<y>"
  Selector6/1 -> Bus Selector6/1
  Bus Selector7/1 -> Mux/7  "<x>"
  Bus Selector7/2 -> Mux1/7  "<y>"
  Selector7/1 -> Bus Selector7/1
  Bus Selector8/1 -> Mux/8  "<x>"
  Bus Selector8/2 -> Mux1/8  "<y>"
  Selector8/1 -> Bus Selector8/1
  Bus Selector9/1 -> Mux/9  "<x>"
  Bus Selector9/2 -> Mux1/9  "<y>"
  Selector9/1 -> Bus Selector9/1
  Bus Selector10/1 -> Mux/10  "<x>"
  Bus Selector10/2 -> Mux1/10  "<y>"
  Selector10/1 -> Bus Selector10/1
  Mux/1 -> x/1
  Mux1/1 -> y/1

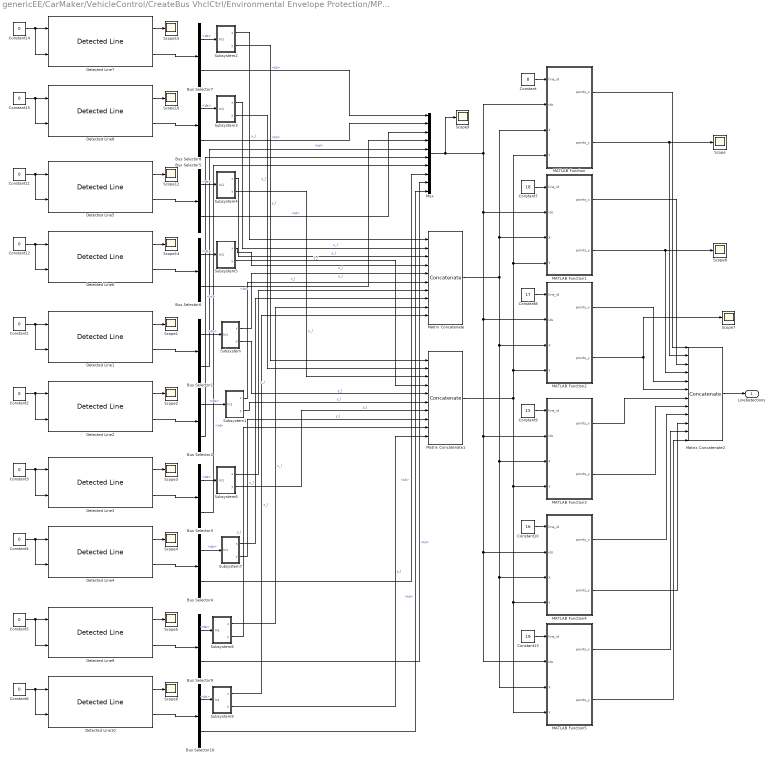
== system genericEE/CarMaker/VehicleControl/CreateBus VhclCtrl/Environmental Envelope Protection/MPC/for ruts ==
  Bus Selector{1..10} (10 alike) : BusSelector  OutputSignals=ds,Id
  Constant : Constant  Value=8
  Constant{1..6,11..12,14..15} (10 alike) : Constant  Value=0
  Constant10 : Constant  Value=16
  Constant13 : Constant  Value=19
  Constant7 : Constant  Value=18
  Constant8 : Constant  Value=17
  Constant9 : Constant  Value=15
  Detected Line1 : CarMaker4SL/Sensors/Detected Line  xname=LS3  xstime=Continuous  xside=left
      settings: SourceProductName=CarMaker4SL
  Detected Line10 : CarMaker4SL/Sensors/Detected Line  xname=LS5  xstime=Continuous  xside=right
      settings: SourceProductName=CarMaker4SL
  Detected Line2 : CarMaker4SL/Sensors/Detected Line  xname=LS3  xstime=Continuous  xside=right
      settings: SourceProductName=CarMaker4SL
  Detected Line3 : CarMaker4SL/Sensors/Detected Line  xname=LS4  xstime=Continuous  xside=left
      settings: SourceProductName=CarMaker4SL
  Detected Line4 : CarMaker4SL/Sensors/Detected Line  xname=LS4  xstime=Continuous  xside=right
      settings: SourceProductName=CarMaker4SL
  Detected Line5 : CarMaker4SL/Sensors/Detected Line  xname=LS2  xstime=Continuous  xside=left
      settings: SourceProductName=CarMaker4SL
  Detected Line6 : CarMaker4SL/Sensors/Detected Line  xname=LS2  xstime=Continuous  xside=right
      settings: SourceProductName=CarMaker4SL
  Detected Line7 : CarMaker4SL/Sensors/Detected Line  xname=LS1  xstime=Continuous  xside=left
      settings: SourceProductName=CarMaker4SL
  Detected Line8 : CarMaker4SL/Sensors/Detected Line  xname=LS1  xstime=Continuous  xside=right
      settings: SourceProductName=CarMaker4SL
  Detected Line9 : CarMaker4SL/Sensors/Detected Line  xname=LS5  xstime=Continuous  xside=left
      settings: SourceProductName=CarMaker4SL
  MATLAB Function : MATLAB Function  TreatAsAtomicUnit=on
  MATLAB Function1 : MATLAB Function  TreatAsAtomicUnit=on
  MATLAB Function2 : MATLAB Function  TreatAsAtomicUnit=on
  MATLAB Function3 : MATLAB Function  TreatAsAtomicUnit=on
  MATLAB Function4 : MATLAB Function  TreatAsAtomicUnit=on
  MATLAB Function5 : MATLAB Function  TreatAsAtomicUnit=on
  Matrix Concatenate : Concatenate  NumInputs=10  Mode=Multidimensional array  ConcatenateDimension=2
  Matrix Concatenate1 : Concatenate  NumInputs=10  Mode=Multidimensional array  ConcatenateDimension=2
  Matrix Concatenate2 : Concatenate  NumInputs=12  Mode=Multidimensional array  ConcatenateDimension=2
  Mux : Mux  Inputs=10
  Scope{,1..9,12,14..16} (14 alike) : Scope
  Subsystem : Subsystem
  Subsystem1 : Subsystem
  Subsystem2 : Subsystem
  Subsystem3 : Subsystem
  Subsystem4 : Subsystem
  Subsystem5 : Subsystem
  Subsystem6 : Subsystem
  Subsystem7 : Subsystem
  Subsystem8 : Subsystem
  Subsystem9 : Subsystem
  LineDetections : Outport
  wires:
  Detected Line5/1 -> Scope12/1
  Constant12/1 -> Detected Line6/2, Detected Line6/1
  Detected Line6/2 -> Bus Selector6/1
  Constant14/1 -> Detected Line7/2, Detected Line7/1
  Constant11/1 -> Detected Line5/2, Detected Line5/1
  Detected Line5/2 -> Bus Selector5/1
  Constant15/1 -> Detected Line8/2, Detected Line8/1
  Detected Line7/1 -> Scope15/1
  Detected Line6/1 -> Scope14/1
  Detected Line8/2 -> Bus Selector8/1
  Detected Line7/2 -> Bus Selector7/1
  Detected Line8/1 -> Scope16/1
  Detected Line1/2 -> Bus Selector1/1
  Detected Line2/2 -> Bus Selector2/1
  Constant1/1 -> Detected Line1/2, Detected Line1/1
  Detected Line2/1 -> Scope2/1
  Detected Line1/1 -> Scope1/1
  Constant2/1 -> Detected Line2/2, Detected Line2/1
  Detected Line3/2 -> Bus Selector3/1
  Detected Line4/2 -> Bus Selector4/1
  Constant3/1 -> Detected Line3/2, Detected Line3/1
  Detected Line4/1 -> Scope4/1
  Detected Line3/1 -> Scope3/1
  Constant4/1 -> Detected Line4/2, Detected Line4/1
  Detected Line9/2 -> Bus Selector9/1
  Detected Line10/2 -> Bus Selector10/1
  Constant5/1 -> Detected Line9/2, Detected Line9/1
  Detected Line10/1 -> Scope6/1
  Detected Line9/1 -> Scope5/1
  Constant6/1 -> Detected Line10/2, Detected Line10/1
  Bus Selector1/1 -> Subsystem/1(In1)  "<ds>"
  Bus Selector2/1 -> Subsystem1/1(In1)  "<ds>"
  Bus Selector7/1 -> Subsystem2/1(In1)  "<ds>"
  Bus Selector8/1 -> Subsystem3/1(In1)  "<ds>"
  Bus Selector5/1 -> Subsystem4/1(In1)  "<ds>"
  Bus Selector6/1 -> Subsystem5/1(In1)  "<ds>"
  Bus Selector3/1 -> Subsystem6/1(In1)  "<ds>"
  Bus Selector4/1 -> Subsystem7/1(In1)  "<ds>"
  Bus Selector9/1 -> Subsystem8/1(In1)  "<ds>"
  Bus Selector10/1 -> Subsystem9/1(In1)  "<ds>"
  Bus Selector7/2 -> Mux/1  "<Id>"
  Bus Selector8/2 -> Mux/2  "<Id>"
  Bus Selector5/2 -> Mux/3  "<Id>"
  Bus Selector6/2 -> Mux/4  "<Id>"
  Bus Selector1/2 -> Mux/5  "<Id>"
  Bus Selector2/2 -> Mux/6  "<Id>"
  Bus Selector3/2 -> Mux/7  "<Id>"
  Bus Selector4/2 -> Mux/8  "<Id>"
  Bus Selector9/2 -> Mux/9  "<Id>"
  Bus Selector10/2 -> Mux/10  "<Id>"
  Subsystem2/1(x) -> Matrix Concatenate/1  "x_l"
  Subsystem3/1(x) -> Matrix Concatenate/2  "x_l"
  Subsystem4/1(x) -> Matrix Concatenate/3  "x_l"
  Subsystem5/1(x) -> Matrix Concatenate/4  "x_l"
  Subsystem/1(x) -> Matrix Concatenate/5  "x_l"
  Subsystem1/1(x) -> Matrix Concatenate/6  "x_l"
  Subsystem6/1(x) -> Matrix Concatenate/7  "x_l"
  Subsystem7/1(x) -> Matrix Concatenate/8  "x_l"
  Subsystem8/1(x) -> Matrix Concatenate/9  "x_l"
  Subsystem9/1(x) -> Matrix Concatenate/10  "x_l"
  Subsystem2/2(y) -> Matrix Concatenate1/1  "y_l"
  Subsystem3/2(y) -> Matrix Concatenate1/2  "y_l"
  Subsystem4/2(y) -> Matrix Concatenate1/3  "y_l"
  Subsystem5/2(y) -> Matrix Concatenate1/4  "y_l"
  Subsystem/2(y) -> Matrix Concatenate1/5  "y_l"
  Subsystem1/2(y) -> Matrix Concatenate1/6  "y_l"
  Subsystem6/2(y) -> Matrix Concatenate1/7  "y_l"
  Subsystem7/2(y) -> Matrix Concatenate1/8  "y_l"
  Subsystem8/2(y) -> Matrix Concatenate1/9  "y_l"
  Subsystem9/2(y) -> Matrix Concatenate1/10  "y_l"
  Constant/1 -> MATLAB Function/1(line_id)
  MATLAB Function1/1(points_x) -> Matrix Concatenate2/3
  MATLAB Function1/2(points_y) -> Scope8/1, Matrix Concatenate2/4
  Constant7/1 -> MATLAB Function1/1(line_id)
  MATLAB Function/1(points_x) -> Matrix Concatenate2/1
  MATLAB Function/2(points_y) -> Matrix Concatenate2/2, Scope/1
  Constant8/1 -> MATLAB Function2/1(line_id)
  Constant9/1 -> MATLAB Function3/1(line_id)
  Constant10/1 -> MATLAB Function4/1(line_id)
  Matrix Concatenate/1 -> MATLAB Function5/3(X), MATLAB Function4/3(X), MATLAB Function3/3(X), MATLAB Function2/3(X), MATLAB Function1/3(X), MATLAB Function/3(X)
  Constant13/1 -> MATLAB Function5/1(line_id)
  Mux/1 -> Scope9/1, MATLAB Function/2(ids), MATLAB Function5/2(ids), MATLAB Function4/2(ids), MATLAB Function3/2(ids), MATLAB Function2/2(ids), MATLAB Function1/2(ids)
  Matrix Concatenate1/1 -> MATLAB Function5/4(Y), MATLAB Function4/4(Y), MATLAB Function3/4(Y), MATLAB Function2/4(Y), MATLAB Function/4(Y), MATLAB Function1/4(Y)
  MATLAB Function2/1(points_x) -> Matrix Concatenate2/5
  MATLAB Function2/2(points_y) -> Scope7/1, Matrix Concatenate2/6
  MATLAB Function3/1(points_x) -> Matrix Concatenate2/7
  MATLAB Function3/2(points_y) -> Matrix Concatenate2/8
  MATLAB Function4/1(points_x) -> Matrix Concatenate2/9
  MATLAB Function4/2(points_y) -> Matrix Concatenate2/10
  MATLAB Function5/1(points_x) -> Matrix Concatenate2/11
  MATLAB Function5/2(points_y) -> Matrix Concatenate2/12
  Matrix Concatenate2/1 -> LineDetections/1

== system genericEE/CarMaker/VehicleControl/CreateBus VhclCtrl/Environmental Envelope Protection/MPC/for ruts/Subsystem ==
  In1 : Inport
  Bus Selector{1..10} (10 alike) : BusSelector  OutputSignals=x,y,z
  Mux : Mux  Inputs=10
  Mux1 : Mux  Inputs=10
  Selector1 : Selector  InputPortWidth=200  IndexOptions=Index vector (dialog)  Indices=1  OutputSizes=1
  Selector10 : Selector  InputPortWidth=200  IndexOptions=Index vector (dialog)  Indices=10  OutputSizes=1
  Selector2 : Selector  InputPortWidth=200  IndexOptions=Index vector (dialog)  Indices=2  OutputSizes=1
  Selector3 : Selector  InputPortWidth=200  IndexOptions=Index vector (dialog)  Indices=3  OutputSizes=1
  Selector4 : Selector  InputPortWidth=200  IndexOptions=Index vector (dialog)  Indices=4  OutputSizes=1
  Selector5 : Selector  InputPortWidth=200  IndexOptions=Index vector (dialog)  Indices=5  OutputSizes=1
  Selector6 : Selector  InputPortWidth=200  IndexOptions=Index vector (dialog)  Indices=6  OutputSizes=1
  Selector7 : Selector  InputPortWidth=200  IndexOptions=Index vector (dialog)  Indices=7  OutputSizes=1
  Selector8 : Selector  InputPortWidth=200  IndexOptions=Index vector (dialog)  Indices=8  OutputSizes=1
  Selector9 : Selector  InputPortWidth=200  IndexOptions=Index vector (dialog)  Indices=9  OutputSizes=1
  x : Outport
  y : Outport  Port=2
  wires:
  Bus Selector1/1 -> Mux/1  "<x>"
  Bus Selector2/2 -> Mux1/2  "<y>"
  In1/1 -> Selector2/1, Selector10/1, Selector9/1, Selector8/1, Selector7/1, Selector6/1, Selector5/1, Selector4/1, Selector3/1, Selector1/1
  Bus Selector2/1 -> Mux/2  "<x>"
  Selector2/1 -> Bus Selector2/1
  Selector1/1 -> Bus Selector1/1
  Bus Selector1/2 -> Mux1/1  "<y>"
  Bus Selector3/1 -> Mux/3  "<x>"
  Bus Selector3/2 -> Mux1/3  "<y>"
  Selector3/1 -> Bus Selector3/1
  Bus Selector4/1 -> Mux/4  "<x>"
  Bus Selector4/2 -> Mux1/4  "<y>"
  Selector4/1 -> Bus Selector4/1
  Bus Selector5/1 -> Mux/5  "<x>"
  Bus Selector5/2 -> Mux1/5  "<y>"
  Selector5/1 -> Bus Selector5/1
  Bus Selector6/1 -> Mux/6  "<x>"
  Bus Selector6/2 -> Mux1/6  "<y>"
  Selector6/1 -> Bus Selector6/1
  Bus Selector7/1 -> Mux/7  "<x>"
  Bus Selector7/2 -> Mux1/7  "<y>"
  Selector7/1 -> Bus Selector7/1
  Bus Selector8/1 -> Mux/8  "<x>"
  Bus Selector8/2 -> Mux1/8  "<y>"
  Selector8/1 -> Bus Selector8/1
  Bus Selector9/1 -> Mux/9  "<x>"
  Bus Selector9/2 -> Mux1/9  "<y>"
  Selector9/1 -> Bus Selector9/1
  Bus Selector10/1 -> Mux/10  "<x>"
  Bus Selector10/2 -> Mux1/10  "<y>"
  Selector10/1 -> Bus Selector10/1
  Mux1/1 -> y/1
  Mux/1 -> x/1

== system genericEE/CarMaker/VehicleControl/CreateBus VhclCtrl/Environmental Envelope Protection/MPC/for ruts/Subsystem1 ==
  In1 : Inport
  Bus Selector{1..10} (10 alike) : BusSelector  OutputSignals=x,y,z
  Mux : Mux  Inputs=10
  Mux1 : Mux  Inputs=10
  Selector1 : Selector  InputPortWidth=200  IndexOptions=Index vector (dialog)  Indices=1  OutputSizes=1
  Selector10 : Selector  InputPortWidth=200  IndexOptions=Index vector (dialog)  Indices=10  OutputSizes=1
  Selector2 : Selector  InputPortWidth=200  IndexOptions=Index vector (dialog)  Indices=2  OutputSizes=1
  Selector3 : Selector  InputPortWidth=200  IndexOptions=Index vector (dialog)  Indices=3  OutputSizes=1
  Selector4 : Selector  InputPortWidth=200  IndexOptions=Index vector (dialog)  Indices=4  OutputSizes=1
  Selector5 : Selector  InputPortWidth=200  IndexOptions=Index vector (dialog)  Indices=5  OutputSizes=1
  Selector6 : Selector  InputPortWidth=200  IndexOptions=Index vector (dialog)  Indices=6  OutputSizes=1
  Selector7 : Selector  InputPortWidth=200  IndexOptions=Index vector (dialog)  Indices=7  OutputSizes=1
  Selector8 : Selector  InputPortWidth=200  IndexOptions=Index vector (dialog)  Indices=8  OutputSizes=1
  Selector9 : Selector  InputPortWidth=200  IndexOptions=Index vector (dialog)  Indices=9  OutputSizes=1
  x : Outport
  y : Outport  Port=2
  wires:
  Bus Selector1/1 -> Mux/1  "<x>"
  Bus Selector2/2 -> Mux1/2  "<y>"
  In1/1 -> Selector2/1, Selector10/1, Selector9/1, Selector8/1, Selector7/1, Selector6/1, Selector5/1, Selector4/1, Selector3/1, Selector1/1
  Bus Selector2/1 -> Mux/2  "<x>"
  Selector2/1 -> Bus Selector2/1
  Selector1/1 -> Bus Selector1/1
  Bus Selector1/2 -> Mux1/1  "<y>"
  Bus Selector3/1 -> Mux/3  "<x>"
  Bus Selector3/2 -> Mux1/3  "<y>"
  Selector3/1 -> Bus Selector3/1
  Bus Selector4/1 -> Mux/4  "<x>"
  Bus Selector4/2 -> Mux1/4  "<y>"
  Selector4/1 -> Bus Selector4/1
  Bus Selector5/1 -> Mux/5  "<x>"
  Bus Selector5/2 -> Mux1/5  "<y>"
  Selector5/1 -> Bus Selector5/1
  Bus Selector6/1 -> Mux/6  "<x>"
  Bus Selector6/2 -> Mux1/6  "<y>"
  Selector6/1 -> Bus Selector6/1
  Bus Selector7/1 -> Mux/7  "<x>"
  Bus Selector7/2 -> Mux1/7  "<y>"
  Selector7/1 -> Bus Selector7/1
  Bus Selector8/1 -> Mux/8  "<x>"
  Bus Selector8/2 -> Mux1/8  "<y>"
  Selector8/1 -> Bus Selector8/1
  Bus Selector9/1 -> Mux/9  "<x>"
  Bus Selector9/2 -> Mux1/9  "<y>"
  Selector9/1 -> Bus Selector9/1
  Bus Selector10/1 -> Mux/10  "<x>"
  Bus Selector10/2 -> Mux1/10  "<y>"
  Selector10/1 -> Bus Selector10/1
  Mux1/1 -> y/1
  Mux/1 -> x/1

== system genericEE/CarMaker/VehicleControl/CreateBus VhclCtrl/Environmental Envelope Protection/MPC/for ruts/Subsystem2 ==
  In1 : Inport
  Bus Selector{1..10} (10 alike) : BusSelector  OutputSignals=x,y,z
  Mux : Mux  Inputs=10
  Mux1 : Mux  Inputs=10
  Selector1 : Selector  InputPortWidth=200  IndexOptions=Index vector (dialog)  Indices=1  OutputSizes=1
  Selector10 : Selector  InputPortWidth=200  IndexOptions=Index vector (dialog)  Indices=10  OutputSizes=1
  Selector2 : Selector  InputPortWidth=200  IndexOptions=Index vector (dialog)  Indices=2  OutputSizes=1
  Selector3 : Selector  InputPortWidth=200  IndexOptions=Index vector (dialog)  Indices=3  OutputSizes=1
  Selector4 : Selector  InputPortWidth=200  IndexOptions=Index vector (dialog)  Indices=4  OutputSizes=1
  Selector5 : Selector  InputPortWidth=200  IndexOptions=Index vector (dialog)  Indices=5  OutputSizes=1
  Selector6 : Selector  InputPortWidth=200  IndexOptions=Index vector (dialog)  Indices=6  OutputSizes=1
  Selector7 : Selector  InputPortWidth=200  IndexOptions=Index vector (dialog)  Indices=7  OutputSizes=1
  Selector8 : Selector  InputPortWidth=200  IndexOptions=Index vector (dialog)  Indices=8  OutputSizes=1
  Selector9 : Selector  InputPortWidth=200  IndexOptions=Index vector (dialog)  Indices=9  OutputSizes=1
  x : Outport
  y : Outport  Port=2
  wires:
  Bus Selector1/1 -> Mux/1  "<x>"
  Bus Selector2/2 -> Mux1/2  "<y>"
  In1/1 -> Selector2/1, Selector10/1, Selector9/1, Selector8/1, Selector7/1, Selector6/1, Selector5/1, Selector4/1, Selector3/1, Selector1/1
  Bus Selector2/1 -> Mux/2  "<x>"
  Selector2/1 -> Bus Selector2/1
  Selector1/1 -> Bus Selector1/1
  Bus Selector1/2 -> Mux1/1  "<y>"
  Bus Selector3/1 -> Mux/3  "<x>"
  Bus Selector3/2 -> Mux1/3  "<y>"
  Selector3/1 -> Bus Selector3/1
  Bus Selector4/1 -> Mux/4  "<x>"
  Bus Selector4/2 -> Mux1/4  "<y>"
  Selector4/1 -> Bus Selector4/1
  Bus Selector5/1 -> Mux/5  "<x>"
  Bus Selector5/2 -> Mux1/5  "<y>"
  Selector5/1 -> Bus Selector5/1
  Bus Selector6/1 -> Mux/6  "<x>"
  Bus Selector6/2 -> Mux1/6  "<y>"
  Selector6/1 -> Bus Selector6/1
  Bus Selector7/1 -> Mux/7  "<x>"
  Bus Selector7/2 -> Mux1/7  "<y>"
  Selector7/1 -> Bus Selector7/1
  Bus Selector8/1 -> Mux/8  "<x>"
  Bus Selector8/2 -> Mux1/8  "<y>"
  Selector8/1 -> Bus Selector8/1
  Bus Selector9/1 -> Mux/9  "<x>"
  Bus Selector9/2 -> Mux1/9  "<y>"
  Selector9/1 -> Bus Selector9/1
  Bus Selector10/1 -> Mux/10  "<x>"
  Bus Selector10/2 -> Mux1/10  "<y>"
  Selector10/1 -> Bus Selector10/1
  Mux1/1 -> y/1
  Mux/1 -> x/1
